simulink model "untitled"  (Simulink 6.0)
settings: Solver=ode45  StartTime=0.0  StopTime=10.0  RelTol=1e-3
libraries: fuzblock x1
settings Model: LastModifiedBy=student
settings OptimizationCC: BooleanDataType=off

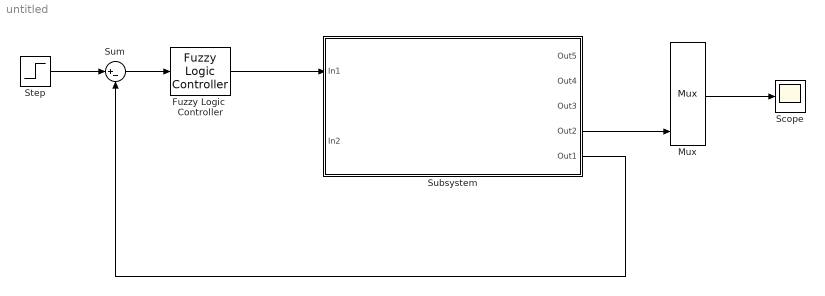
== system untitled ==
  Fuzzy Logic  Controller : fuzblock/Fuzzy Logic  Controller  fis=inferente
  Mux : Mux
  Scope : Scope
  Step : Step  SampleTime=0
  Subsystem : Subsystem
  Sum : Sum  Inputs=|+-
  wires:
  Fuzzy Logic  Controller/1 -> Subsystem/1(In1)
  Sum/1 -> Fuzzy Logic  Controller/1
  Step/1 -> Sum/1
  Subsystem/5(Out1) -> Sum/2
  Mux/1 -> Scope/1
  Subsystem/4(Out2) -> Mux/4

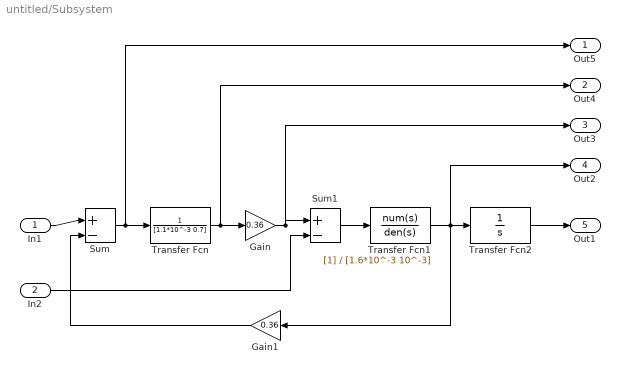
== system untitled/Subsystem ==
  In1 : Inport  Port=1  LatchInput=off
  In2 : Inport  Port=2  LatchInput=off
  Gain : Gain  Gain=0.36
  Gain1 : Gain  Orientation=left  Gain=0.36
  Sum : Sum  Inputs=|+-
  Sum1 : Sum  Inputs=|+-
  Transfer Fcn : TransferFcn  Denominator=[1.1*10^-3 0.7]
  Transfer Fcn1 : TransferFcn  Denominator=[1.6*10^-3 10^-3]
  Transfer Fcn2 : TransferFcn  Denominator=[1 0]
  Out5 : Outport
  Out4 : Outport  Port=2
  Out3 : Outport  Port=3
  Out2 : Outport  Port=4
  Out1 : Outport  Port=5
  wires:
  Sum/1 -> Transfer Fcn/1, Out5/1
  Transfer Fcn/1 -> Gain/1, Out4/1
  Gain/1 -> Sum1/1, Out3/1
  Sum1/1 -> Transfer Fcn1/1
  Transfer Fcn1/1 -> Transfer Fcn2/1, Gain1/1, Out2/1
  In2/1 -> Sum1/2
  Gain1/1 -> Sum/2
  Transfer Fcn2/1 -> Out1/1
  In1/1 -> Sum/1
